simulink model "power_aircraft_distribution"  (R2014b)
settings: Solver=ode4  StartTime=0.0  StopTime=4.5  FixedStep=Ts  RelTol=5e-3
PreLoadFcn:
  | warning off
  | Ts=10e-6;
InitFcn:
  | warning off
  | Ts=10e-6;
StopFcn:
  | warning on
undefined symbols (not defined in the file or in its folder): D1, Delta, driveGuiManager, gcbh, sigbuilder_block
libraries: powerlib x51, simulink x4, simulink_extras x4, AC6DriveInternalModels x3, powerlib_meascontrol x2, DriveInternalModels x1, sps_avr x1
(part 2 of 2)

== system power_aircraft_distribution/AC Load : 2 kW Brushless motor driving a ballscrew actuator/PM Synchronous Motor Drive1/Braking chopper/Proportional controller/Ramp_generator ==
  Constant3 : Constant
  Discrete-Time Integrator1 : DiscreteIntegrator  ExternalReset=rising  SampleTime=Ts
  Relational Operator1 : RelationalOperator  InputSameDT=on
  Unit Delay1 : UnitDelay  SampleTime=Ts
  fc : Constant  Value=freq_chop
  ramp_out : Outport
  wires:
  Unit Delay1/1 -> Discrete-Time Integrator1/2
  Relational Operator1/1 -> Unit Delay1/1
  Constant3/1 -> Relational Operator1/2
  Discrete-Time Integrator1/1 -> ramp_out/1, Relational Operator1/1
  fc/1 -> Discrete-Time Integrator1/1
